simulink model "ExoskeletonControlModel"  (R2022b)
settings: Solver=ode3  StartTime=0.0  StopTime=inf  FixedStep=Ts  RelTol=1e-3
PreLoadFcn:
  | Ts_IO204 = 0.001;
  | 
  | if ~exist('Ts', 'var')
  | Ts = 0.001;
  | end
  | if ~exist('FPGA_Frequency', 'var')
  | FPGA_Frequency = 75000000;
  | end
  | 
  | ts_IO612 = 1e-3;
  | 
  | load('TargetReached.mat')
  | load('ActualPos_inc.mat')
model workspace (MAT data in the model file):
  DeltaData : timeseries (value not decoded)
  EC45_deg2incs = 2276
  EC60_deg2inc = 5461
  EC90_deg2incs = 7111
  Enc2rad_18bit = 2.3968e-05
  Enc2rad_19bit = 1.1984e-05
  Enc2rad_20bit = 5.9921e-06
  GiulioModel : robotics.RigidBodyTree (value not decoded)
  Giulio_Spheric_model : robotics.RigidBodyTree (value not decoded)
  Offset1_ticks = 571315
  Offset2_ticks = 590938.9928
  Offset3_ticks = 457912.8279
  Offset4_ticks = 482293.9763
  Offset5_ticks = 598735.9316
  Offset_M1 = 1.12645499896
  Offset_M2 = 4.02728553608
  Offset_M3 = 5.48587511336
  Offset_M4 = 2.03717511516
  Offset_M5 = 4.4996674016
  T1_Nm : object (value not decoded)
  T2_Nm : object (value not decoded)
  TBmodel : robotics.RigidBodyTree (value not decoded)
  Ts = 0.002
  Xg : object (value not decoded)
  Yg : object (value not decoded)
  Zg : object (value not decoded)
  a2 = 0.27
  change_variable = 0
  d1 = [0 0 0 0 0 0 0 0 0 0 0 0 ... (30001 elements, 30001x1)]
  d1_1 = 0.21074
  d2 = [0 0 0 0 0 0 0 0 0 0 0 0 ... (30001 elements, 30001x1)]
  d2_1 = 0.04864
  d3 = [0 0 0 0 0 0 0 0 0 0 0 0 ... (30001 elements, 30001x1)]
  d4 = [0 0 0 0 0 0 0 0 0 0 0 0 ... (30001 elements, 30001x1)]
  d5 = [0 0 0 0 0 0 0 0 0 0 0 0 ... (30001 elements, 30001x1)]
  d6 = [0 0 0 0 0 0 0 0 0 0 0 0 ... (30001 elements, 30001x1)]
  ee_x = -0.2852
  ee_y = -0.3683
  ee_z = -0.0386
  enc2rad_EC45 = 7.6699e-06
  enc2rad_EC90 = 2.3969e-05
  k1_Nm_ticks = 0.00923
  k2_Nm_ticks = 0.0257
  k3_Nm_ticks = 0.00692
  k4_Nm_ticks = 0.00729
  k5_Nm_ticks = 0.00641
  lower_lim_m1 = -330000
  lower_lim_m2 = -235302
  lower_lim_m3 = -132865
  lower_lim_m4 = -152732
  lower_lim_m5 = -138363
  lower_lim_m6 = -200325
  m1 = 2.441408578
  m2 = 3.750007
  m3 = 1.56250298
  m4 = 1.56250298
  m5 = 1.56250298
  m6 = 1.56250298
  n_oversampling = 8
  offset_sea_1 = 0.5547
  offset_sea_2 = 2.8595
  offset_sea_3 = 3.5058
  offset_sea_4 = 2.8586
  offset_sea_5 = 2.8736
  params : AKSIM (value not decoded)
  pos_th_neg = -180000
  pos_th_pos = 180000
  q1 = -1819347
  q2 = -196752
  q3 = -596465
  q4 = -556807
  q5 = -573932
  q6 = -489063
  sine = [0 0.187999937334 0.751998997352 1.69199492401 3.0079839574 4.6999608335 6.76791878442 9.21184953835 12.0317433196 15.2275888485 18.7993733417 22.7470825122 ... (12501 elements, 12501x1)]
  start : object (value not decoded)
  switch_admittance = 1
  t1 : object (value not decoded)
  t2 : object (value not decoded)
  torsionalStiffnes_M1 = 384.88
  torsionalStiffnes_M2 = 1500
  torsionalStiffnes_M3 = 901.97
  torsionalStiffnes_M4 = 950.86
  torsionalStiffnes_M5 = 930
  torsionalStiffnes_M6 = 914
  upper_lim_m1 = 340000
  upper_lim_m2 = 95467
  upper_lim_m3 = 164951
  upper_lim_m4 = 210607
  upper_lim_m5 = 252595
  upper_lim_m6 = 96694
  vel_th_neg = -100
  vel_th_pos = 100
  x = 0
undefined symbols (not defined in the file): C, DiscIntNeverNeededParam
libraries: canmsglib x285, speedgoatlib_IO614 x245, simulink x26, slrealtimeloglib x9, simulink_extras x6, robotmaniplib x6
(part 4 of 13)

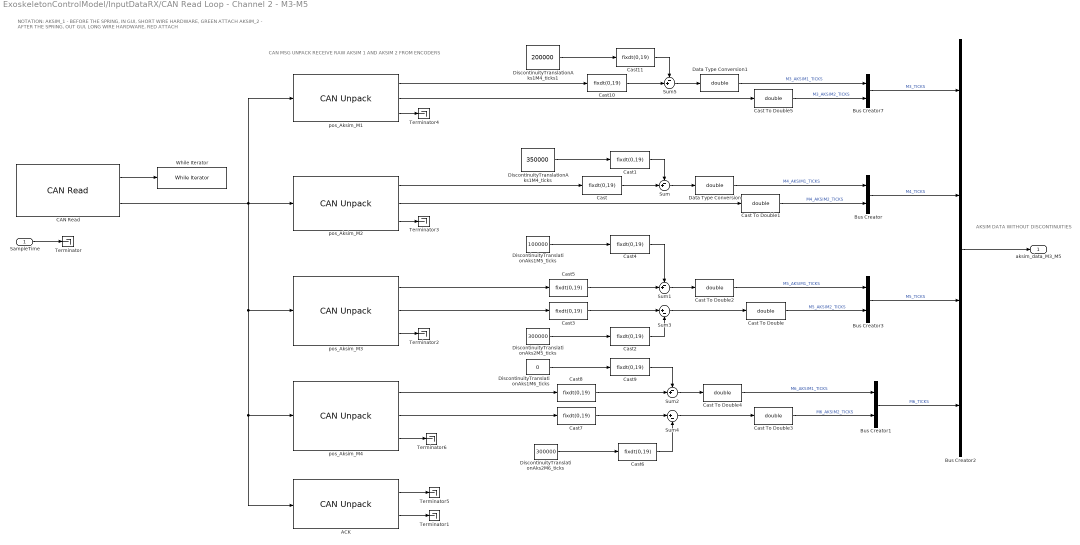
== system ExoskeletonControlModel/InputDataRX/CAN Read Loop - Channel 2 - M3-M5 ==
  note: AKSIM DATA WITHOUT DISCONTINUITIES
  note: CAN MSG UNPACK
      | RECEIVE RAW AKSIM 1 AND AKSIM 2 FROM ENCODERS
  note: NOTATION:
      | AKSIM_1 - BEFORE THE SPRING, IN GUI, SHORT WIRE HARDWARE, GREEN ATTACH
      | AKSIM_2 - AFTER THE SPRING, OUT GUI, LONG WIRE HARDWARE, RED ATTACH
  SampleTime : Inport
  ACK : canmsglib/CAN Unpack  MsgList=(none)  MsgName=CAN Msg  MsgIDType=Standard (11-bit identifier)  MsgIdentifier=hex2dec('10C')  MsgLength=8  SignalInfo={ 'Signal1', '0', '8', 'LE', 'signed', 'Standard', '0', '1', '0', '-Inf', 'Inf' }  IDPort=off  TimestampPort=off  ErrorPort=off  RemotePort=off  LengthPort=off  StatusPort=on  ApplyMinMax=off
  Bus Creator{,1,3,7} (4 alike) : BusCreator  Inputs=2
  Bus Creator2 : BusCreator  Inputs=4
  CAN Read : speedgoatlib_IO614/CAN/CAN Read  id=1  sampleTime=-1  portSelection=2  messageType=CAN  protl=IO614  ptIdx=1  isFDMod=0
  Cast{,1..11} (12 alike) : DataTypeConversion  OutMin=0  OutMax=2^19-1  OutDataTypeStr=fixdt(0,19)  SaturateOnIntegerOverflow=off  RndMeth=Floor
  Cast To Double{,1..5} (6 alike) : DataTypeConversion  OutDataTypeStr=double  SaturateOnIntegerOverflow=off  RndMeth=Floor
  Data Type Conversion : DataTypeConversion  OutDataTypeStr=double  SaturateOnIntegerOverflow=off  RndMeth=Floor
  Data Type Conversion1 : DataTypeConversion  OutDataTypeStr=double  SaturateOnIntegerOverflow=off  RndMeth=Floor
  DiscontinuityTranslationAks1M4_ticks : Constant  Value=350000
  DiscontinuityTranslationAks1M4_ticks1 : Constant  Value=200000
  DiscontinuityTranslationAks1M5_ticks : Constant  Value=100000
  DiscontinuityTranslationAks1M6_ticks : Constant  Value=0
  DiscontinuityTranslationAks2M5_ticks : Constant  Value=300000
  DiscontinuityTranslationAks2M6_ticks : Constant  Value=300000
  Sum{,1..2,5} (4 alike) : Sum  Inputs=-+|  OutDataTypeStr=Inherit: Same as first input
  Sum3 : Sum  Inputs=|+-  OutDataTypeStr=Inherit: Same as first input
  Sum4 : Sum  Inputs=|+-  OutDataTypeStr=Inherit: Same as first input
  Terminator{,1..6} (7 alike) : Terminator
  While Iterator : WhileIterator  MaxIters=501  WhileBlockType=do-while
  pos_Aksim_M1 : canmsglib/CAN Unpack  MsgList=(none)  MsgName=CAN Msg  MsgIDType=Standard (11-bit identifier)  MsgIdentifier=hex2dec('102')  MsgLength=8  SignalInfo={ 'AKSIM_1', '0', '32', 'LE', 'unsigned', 'Standard', '0', '1', '0', '-Inf', 'Inf'; 'AKSIM_2', '32', '32', 'LE', 'unsigned', 'Standard', '0', '1', '0', '-Inf', 'Inf' }  IDPort=off  TimestampPort=off  ErrorPort=off  RemotePort=on  LengthPort=off  StatusPort=off  ApplyMinMax=off
  pos_Aksim_M2 : canmsglib/CAN Unpack  MsgList=(none)  MsgName=CAN Msg  MsgIDType=Standard (11-bit identifier)  MsgIdentifier=hex2dec('202')  MsgLength=8  SignalInfo={ 'AKSIM_1', '0', '32', 'LE', 'unsigned', 'Standard', '0', '1', '0', '-Inf', 'Inf'; 'AKSIM_2', '32', '32', 'LE', 'unsigned', 'Standard', '0', '1', '0', '-Inf', 'Inf' }  IDPort=off  TimestampPort=off  ErrorPort=off  RemotePort=on  LengthPort=off  StatusPort=off  ApplyMinMax=off
  pos_Aksim_M3 : canmsglib/CAN Unpack  MsgList=(none)  MsgName=CAN Msg  MsgIDType=Standard (11-bit identifier)  MsgIdentifier=hex2dec('302')  MsgLength=8  SignalInfo={ 'AKSIM_1', '0', '32', 'LE', 'unsigned', 'Standard', '0', '1', '0', '-Inf', 'Inf'; 'AKSIM_2', '32', '32', 'LE', 'unsigned', 'Standard', '0', '1', '0', '-Inf', 'Inf' }  IDPort=off  TimestampPort=off  ErrorPort=off  RemotePort=on  LengthPort=off  StatusPort=off  ApplyMinMax=off
  pos_Aksim_M4 : canmsglib/CAN Unpack  MsgList=(none)  MsgName=CAN Msg  MsgIDType=Standard (11-bit identifier)  MsgIdentifier=hex2dec('402')  MsgLength=8  SignalInfo={ 'AKSIM_1', '0', '32', 'LE', 'unsigned', 'Standard', '0', '1', '0', '-Inf', 'Inf'; 'AKSIM_2', '32', '32', 'LE', 'unsigned', 'Standard', '0', '1', '0', '-Inf', 'Inf' }  IDPort=off  TimestampPort=off  ErrorPort=off  RemotePort=on  LengthPort=off  StatusPort=off  ApplyMinMax=off
  aksim_data_M3_M5 : Outport
  wires:
  SampleTime/1 -> Terminator/1
  CAN Read/1 -> While Iterator/1
  pos_Aksim_M1/3 -> Terminator4/1
  Cast To Double5/1 -> Bus Creator7/2  "M3_AKSIM2_TICKS"
  ACK/2 -> Terminator1/1
  pos_Aksim_M2/1 -> Cast/1
  ACK/1 -> Terminator5/1
  Data Type Conversion1/1 -> Bus Creator7/1  "M3_AKSIM1_TICKS"
  pos_Aksim_M2/3 -> Terminator3/1
  Bus Creator2/1 -> aksim_data_M3_M5/1
  Bus Creator/1 -> Bus Creator2/2  "M4_TICKS"
  Bus Creator7/1 -> Bus Creator2/1  "M3_TICKS"
  pos_Aksim_M3/1 -> Cast5/1
  Bus Creator3/1 -> Bus Creator2/3  "M5_TICKS"
  pos_Aksim_M3/2 -> Cast3/1
  pos_Aksim_M3/3 -> Terminator2/1
  Sum/1 -> Data Type Conversion/1
  pos_Aksim_M2/2 -> Cast To Double1/1
  Sum3/1 -> Cast To Double/1
  Cast3/1 -> Sum3/1
  DiscontinuityTranslationAks2M5_ticks/1 -> Cast2/1
  DiscontinuityTranslationAks1M4_ticks/1 -> Cast1/1
  Cast/1 -> Sum/2
  Cast1/1 -> Sum/1
  Cast To Double/1 -> Bus Creator3/2  "M5_AKSIM2_TICKS"
  Cast To Double1/1 -> Bus Creator/2  "M4_AKSIM2_TICKS"
  Data Type Conversion/1 -> Bus Creator/1  "M4_AKSIM1_TICKS"
  Cast2/1 -> Sum3/2
  Cast To Double2/1 -> Bus Creator3/1  "M5_AKSIM1_TICKS"
  Sum1/1 -> Cast To Double2/1
  DiscontinuityTranslationAks1M5_ticks/1 -> Cast4/1
  Cast5/1 -> Sum1/2
  Cast4/1 -> Sum1/1
  Cast9/1 -> Sum2/1
  Cast6/1 -> Sum4/2
  Cast8/1 -> Sum2/2
  DiscontinuityTranslationAks1M6_ticks/1 -> Cast9/1
  Cast To Double4/1 -> Bus Creator1/1  "M6_AKSIM1_TICKS"
  Cast To Double3/1 -> Bus Creator1/2  "M6_AKSIM2_TICKS"
  Sum4/1 -> Cast To Double3/1
  DiscontinuityTranslationAks2M6_ticks/1 -> Cast6/1
  pos_Aksim_M4/1 -> Cast8/1
  pos_Aksim_M4/2 -> Cast7/1
  Sum2/1 -> Cast To Double4/1
  Cast7/1 -> Sum4/1
  CAN Read/2 -> pos_Aksim_M3/1, ACK/1, pos_Aksim_M4/1, pos_Aksim_M2/1, pos_Aksim_M1/1
  pos_Aksim_M4/3 -> Terminator6/1
  Bus Creator1/1 -> Bus Creator2/4  "M6_TICKS"
  Cast11/1 -> Sum5/1
  Sum5/1 -> Data Type Conversion1/1
  Cast10/1 -> Sum5/2
  DiscontinuityTranslationAks1M4_ticks1/1 -> Cast11/1
  pos_Aksim_M1/1 -> Cast10/1
  pos_Aksim_M1/2 -> Cast To Double5/1

== system ExoskeletonControlModel/InputDataRX/CAN Read Loop - Channel 3 ==
  note: PDO M1
  note: PDO M2
  note: STATUS MODE M1 M2
  note: CAN MSG FROM EPOS M1 M2
  SampleTime : Inport
  Bus Creator1 : BusCreator  Inputs=3
  Bus Creator2 : BusCreator  Inputs=5
  Bus Creator3 : BusCreator  Inputs=5
  Bus Creator4 : BusCreator  Inputs=9
  Bus Creator5 : BusCreator  Inputs=4
  Bus Creator6 : BusCreator  Inputs=3
  CAN Read : speedgoatlib_IO614/CAN/CAN Read  id=1  sampleTime=-1  portSelection=3  messageType=CAN  protl=IO614  ptIdx=2  isFDMod=0
  Constant : Constant
  Constant1 : Constant
  EMCY : canmsglib/CAN Unpack  MsgList=(none)  MsgName=CAN Msg  MsgIDType=Standard (11-bit identifier)  MsgIdentifier=129  MsgLength=8  SignalInfo={ 'ErrorCode', '0', '16', 'LE', 'unsigned', 'Standard', '0', '1', '0', '-Inf', 'Inf'; 'ErrorReg', '16', '8', 'LE', 'unsigned', 'Standard', '0', '1', '0', '-Inf', 'Inf' }  IDPort=off  TimestampPort=off  ErrorPort=off  RemotePort=off  LengthPort=off  StatusPort=off  ApplyMinMax=off
  EMCY_m2 : canmsglib/CAN Unpack  MsgList=(none)  MsgName=CAN Msg  MsgIDType=Standard (11-bit identifier)  MsgIdentifier=130  MsgLength=8  SignalInfo={ 'ErrorCode', '0', '16', 'LE', 'unsigned', 'Standard', '0', '1', '0', '-Inf', 'Inf'; 'ErrorReg', '16', '8', 'LE', 'unsigned', 'Standard', '0', '1', '0', '-Inf', 'Inf' }  IDPort=off  TimestampPort=off  ErrorPort=off  RemotePort=off  LengthPort=off  StatusPort=off  ApplyMinMax=off
  HEARTBEAT : canmsglib/CAN Unpack  MsgList=(none)  MsgName=CAN Msg  MsgIDType=Standard (11-bit identifier)  MsgIdentifier=hex2dec('701')  MsgLength=1  SignalInfo={ 'NMT_state', '0', '8', 'LE', 'unsigned', 'Standard', '0', '1', '0', '-Inf', 'Inf' }  IDPort=off  TimestampPort=off  ErrorPort=off  RemotePort=off  LengthPort=off  StatusPort=off  ApplyMinMax=off
  HEARTBEAT_m2 : canmsglib/CAN Unpack  MsgList=(none)  MsgName=CAN Msg  MsgIDType=Standard (11-bit identifier)  MsgIdentifier=hex2dec('702')  MsgLength=1  SignalInfo={ 'NMT_state', '0', '8', 'LE', 'unsigned', 'Standard', '0', '1', '0', '-Inf', 'Inf' }  IDPort=off  TimestampPort=off  ErrorPort=off  RemotePort=off  LengthPort=off  StatusPort=off  ApplyMinMax=off
  Terminator : Terminator
  Terminator1 : Terminator
  Terminator2 : Terminator
  TxPDO1 : canmsglib/CAN Unpack  MsgList=(none)  MsgName=CAN Msg  MsgIDType=Standard (11-bit identifier)  MsgIdentifier=hex2dec('181')  MsgLength=7  SignalInfo={ 'Statusword', '0', '16', 'LE', 'unsigned', 'Standard', '0', '1', '0', '-Inf', 'Inf'; 'Modes Operation', '16', '8', 'LE', 'unsigned', 'Standard', '0', '1', '0', '-Inf', 'Inf'; 'Current actual', '24', '32', 'LE', 'signed', 'Standard', '0', '1', '0', '-Inf', 'Inf' }  IDPort=off  TimestampPort=off  ErrorPort=off  RemotePort=off  LengthPort=off  StatusPort=off  ApplyMinMax=off
  TxPDO1_m2 : canmsglib/CAN Unpack  MsgList=(none)  MsgName=CAN Msg  MsgIDType=Standard (11-bit identifier)  MsgIdentifier=hex2dec('182')  MsgLength=7  SignalInfo={ 'Statusword', '0', '16', 'LE', 'unsigned', 'Standard', '0', '1', '0', '-Inf', 'Inf'; 'Modes Operation', '16', '8', 'LE', 'unsigned', 'Standard', '0', '1', '0', '-Inf', 'Inf'; 'Current actual', '24', '32', 'LE', 'signed', 'Standard', '0', '1', '0', '-Inf', 'Inf' }  IDPort=off  TimestampPort=off  ErrorPort=off  RemotePort=off  LengthPort=off  StatusPort=off  ApplyMinMax=off
  TxPDO2 : canmsglib/CAN Unpack  MsgList=(none)  MsgName=CAN Msg  MsgIDType=Standard (11-bit identifier)  MsgIdentifier=hex2dec('281')  MsgLength=4  SignalInfo={ 'Pos Actual', '0', '32', 'LE', 'signed', 'Standard', '0', '1', '0', '-Inf', 'Inf' }  IDPort=off  TimestampPort=off  ErrorPort=off  RemotePort=off  LengthPort=off  StatusPort=off  ApplyMinMax=off
  TxPDO2_m2 : canmsglib/CAN Unpack  MsgList=(none)  MsgName=CAN Msg  MsgIDType=Standard (11-bit identifier)  MsgIdentifier=hex2dec('282')  MsgLength=4  SignalInfo={ 'Pos Actual', '0', '32', 'LE', 'signed', 'Standard', '0', '1', '0', '-Inf', 'Inf' }  IDPort=off  TimestampPort=off  ErrorPort=off  RemotePort=off  LengthPort=off  StatusPort=off  ApplyMinMax=off
  TxPDO4 : canmsglib/CAN Unpack  MsgList=(none)  MsgName=CAN Msg  MsgIDType=Standard (11-bit identifier)  MsgIdentifier=hex2dec('481')  MsgLength=8  SignalInfo={ 'Velocity Actual Value', '0', '32', 'LE', 'signed', 'Standard', '0', '1', '0', '-Inf', 'Inf'; 'Torque Actual', '32', '16', 'LE', 'signed', 'Standard', '0', '1', '0', '-Inf', 'Inf'; 'Torque Actual Averaged', '48', '16', 'LE', 'signed', 'Standard', '0', '1', '0', '-Inf', 'Inf' }  IDPort=off  TimestampPort=off  ErrorPort=off  RemotePort=off  LengthPort=off  StatusPort=off  ApplyMinMax=off
  TxPDO4_m2 : canmsglib/CAN Unpack  MsgList=(none)  MsgName=CAN Msg  MsgIDType=Standard (11-bit identifier)  MsgIdentifier=hex2dec('482')  MsgLength=8  SignalInfo={ 'Velocity Actual Value', '0', '32', 'LE', 'signed', 'Standard', '0', '1', '0', '-Inf', 'Inf'; 'Torque Actual', '32', '16', 'LE', 'signed', 'Standard', '0', '1', '0', '-Inf', 'Inf'; 'Torque Actual Averaged', '48', '16', 'LE', 'signed', 'Standard', '0', '1', '0', '-Inf', 'Inf' }  IDPort=off  TimestampPort=off  ErrorPort=off  RemotePort=off  LengthPort=off  StatusPort=off  ApplyMinMax=off
  While Iterator : WhileIterator  MaxIters=501  WhileBlockType=do-while
  txSDO : canmsglib/CAN Unpack  MsgList=(none)  MsgName=CAN Msg  MsgIDType=Standard (11-bit identifier)  MsgIdentifier=1409  MsgLength=8  SignalInfo={ 'data', '32', '32', 'LE', 'signed', 'Standard', '0', '1', '0', '-Inf', 'Inf'; 'Index', '8', '16', 'LE', 'unsigned', 'Standard', '0', '1', '0', '-Inf', 'Inf'; 'SubIndex', '24', '8', 'LE', 'unsigned', 'Standard', '0', '1', '0', '-Inf', 'Inf' }  IDPort=off  TimestampPort=off  ErrorPort=off  RemotePort=off  LengthPort=off  StatusPort=off  ApplyMinMax=off
  txSDO1 : canmsglib/CAN Unpack  MsgList=(none)  MsgName=CAN Msg  MsgIDType=Standard (11-bit identifier)  MsgIdentifier=1410  MsgLength=8  SignalInfo={ 'data', '32', '32', 'LE', 'signed', 'Standard', '0', '1', '0', '-Inf', 'Inf'; 'Index', '8', '16', 'LE', 'unsigned', 'Standard', '0', '1', '0', '-Inf', 'Inf'; 'SubIndex', '24', '8', 'LE', 'unsigned', 'Standard', '0', '1', '0', '-Inf', 'Inf' }  IDPort=off  TimestampPort=off  ErrorPort=off  RemotePort=off  LengthPort=off  StatusPort=off  ApplyMinMax=off
  txSDO2 : canmsglib/CAN Unpack  MsgList=(none)  MsgName=CAN Msg  MsgIDType=Standard (11-bit identifier)  MsgIdentifier=1411  MsgLength=8  SignalInfo={ 'data', '32', '32', 'LE', 'signed', 'Standard', '0', '1', '0', '-Inf', 'Inf'; 'Index', '8', '16', 'LE', 'unsigned', 'Standard', '0', '1', '0', '-Inf', 'Inf'; 'SubIndex', '24', '8', 'LE', 'unsigned', 'Standard', '0', '1', '0', '-Inf', 'Inf' }  IDPort=off  TimestampPort=off  ErrorPort=off  RemotePort=off  LengthPort=off  StatusPort=off  ApplyMinMax=off
  SDOs : Outport
  emcy : Outport  Port=2
  NMT_state : Outport  Port=3
  status_mode_m1_m2 : Outport  Port=4
  PDO_m1 : Outport  Port=5
  PDO_m2 : Outport  Port=6
  wires:
  SampleTime/1 -> Terminator/1
  Bus Creator4/1 -> SDOs/1
  txSDO/3 -> Bus Creator4/3  "SDO_subIndex"
  EMCY/2 -> Terminator1/1
  EMCY/1 -> Bus Creator1/1  "error_code_m1"
  Bus Creator1/1 -> emcy/1
  HEARTBEAT/1 -> Bus Creator6/1  "NMT_state_1"
  txSDO/1 -> Bus Creator4/1  "SDO_data"
  txSDO/2 -> Bus Creator4/2  "SDO_index"
  TxPDO1/1 -> Bus Creator5/1  "statusword_1"
  TxPDO1/2 -> Bus Creator5/2  "mode_1"
  TxPDO1/3 -> Bus Creator2/1  "current_actual_1"
  TxPDO2/1 -> Bus Creator2/2  "pos_actual_1"
  TxPDO4/1 -> Bus Creator2/3  "velocity_actual_1"
  TxPDO4/2 -> Bus Creator2/4  "torque_actual_1"
  TxPDO1_m2/3 -> Bus Creator3/1  "current_actual_2"
  TxPDO4_m2/2 -> Bus Creator3/4  "torque_actual_2"
  TxPDO4_m2/1 -> Bus Creator3/3  "velocity_actual_2"
  TxPDO1_m2/2 -> Bus Creator5/4  "mode_2"
  TxPDO2_m2/1 -> Bus Creator3/2  "pos_actual_2"
  TxPDO1_m2/1 -> Bus Creator5/3  "statusword_2"
  Bus Creator2/1 -> PDO_m1/1
  Bus Creator3/1 -> PDO_m2/1
  Bus Creator5/1 -> status_mode_m1_m2/1
  EMCY_m2/1 -> Bus Creator1/2  "error_code_m2"
  EMCY_m2/2 -> Terminator2/1
  HEARTBEAT_m2/1 -> Bus Creator6/2  "NMT_state_2"
  Bus Creator6/1 -> NMT_state/1
  TxPDO4/3 -> Bus Creator2/5  "torque_averaged_1"
  TxPDO4_m2/3 -> Bus Creator3/5  "torque_averaged_2"
  txSDO1/1 -> Bus Creator4/4  "SDO_data2"
  txSDO1/2 -> Bus Creator4/5  "SDO_index2"
  txSDO1/3 -> Bus Creator4/6  "SDO_subIndex2"
  txSDO2/2 -> Bus Creator4/8  "SDO_index3"
  txSDO2/3 -> Bus Creator4/9  "SDO_subIndex3"
  txSDO2/1 -> Bus Creator4/7  "SDO_data3"
  CAN Read/1 -> While Iterator/1
  CAN Read/2 -> txSDO/1, txSDO1/1, txSDO2/1, EMCY_m2/1, HEARTBEAT_m2/1, TxPDO1/1, TxPDO2/1, TxPDO4/1, TxPDO1_m2/1, TxPDO2_m2/1, TxPDO4_m2/1, HEARTBEAT/1, EMCY/1
  Constant/1 -> Bus Creator1/3  "future"
  Constant1/1 -> Bus Creator6/3  "future_NMT"

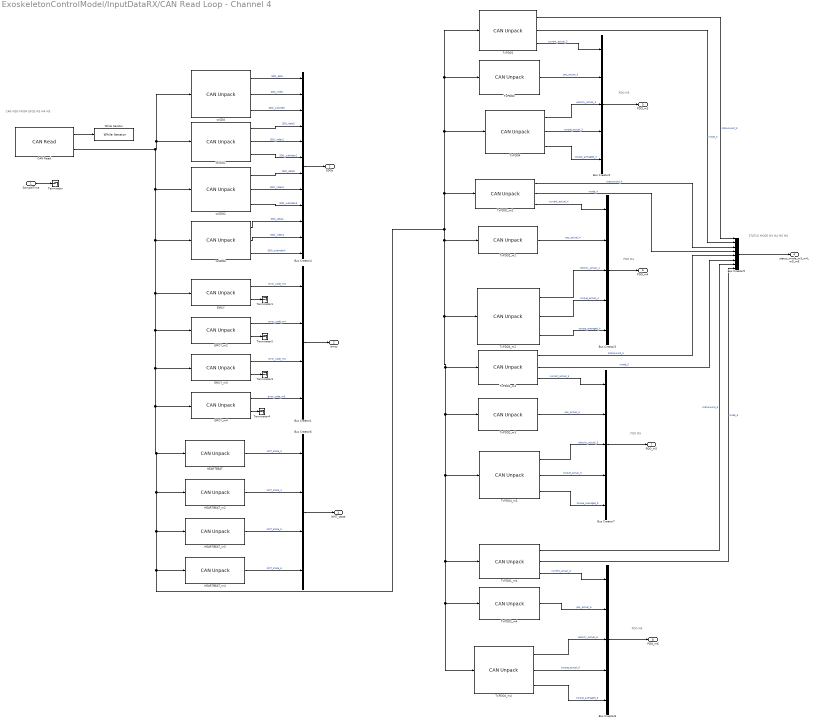
== system ExoskeletonControlModel/InputDataRX/CAN Read Loop - Channel 4 ==
  note: STATUS MODE M3 M4 M5 M6
  note: CAN MSG FROM EPOS M3 M4 M5
  note: PDO M3
  note: PDO M5
  note: PDO M4
  note: PDO M6
  SampleTime : Inport
  Bus Creator1 : BusCreator  Inputs=4
  Bus Creator{2..3,7..8} (4 alike) : BusCreator  Inputs=5
  Bus Creator4 : BusCreator  Inputs=12
  Bus Creator5 : BusCreator  Inputs=8
  Bus Creator6 : BusCreator  Inputs=4
  CAN Read : speedgoatlib_IO614/CAN/CAN Read  id=1  sampleTime=-1  portSelection=4  messageType=CAN  protl=IO614  ptIdx=3  isFDMod=0
  EMCY : canmsglib/CAN Unpack  MsgList=(none)  MsgName=CAN Msg  MsgIDType=Standard (11-bit identifier)  MsgIdentifier=129  MsgLength=8  SignalInfo={ 'ErrorCode', '0', '16', 'LE', 'unsigned', 'Standard', '0', '1', '0', '-Inf', 'Inf'; 'ErrorReg', '16', '8', 'LE', 'unsigned', 'Standard', '0', '1', '0', '-Inf', 'Inf' }  IDPort=off  TimestampPort=off  ErrorPort=off  RemotePort=off  LengthPort=off  StatusPort=off  ApplyMinMax=off
  EMCY_m2 : canmsglib/CAN Unpack  MsgList=(none)  MsgName=CAN Msg  MsgIDType=Standard (11-bit identifier)  MsgIdentifier=130  MsgLength=8  SignalInfo={ 'ErrorCode', '0', '16', 'LE', 'unsigned', 'Standard', '0', '1', '0', '-Inf', 'Inf'; 'ErrorReg', '16', '8', 'LE', 'unsigned', 'Standard', '0', '1', '0', '-Inf', 'Inf' }  IDPort=off  TimestampPort=off  ErrorPort=off  RemotePort=off  LengthPort=off  StatusPort=off  ApplyMinMax=off
  EMCY_m3 : canmsglib/CAN Unpack  MsgList=(none)  MsgName=CAN Msg  MsgIDType=Standard (11-bit identifier)  MsgIdentifier=131  MsgLength=8  SignalInfo={ 'ErrorCode', '0', '16', 'LE', 'unsigned', 'Standard', '0', '1', '0', '-Inf', 'Inf'; 'ErrorReg', '16', '8', 'LE', 'unsigned', 'Standard', '0', '1', '0', '-Inf', 'Inf' }  IDPort=off  TimestampPort=off  ErrorPort=off  RemotePort=off  LengthPort=off  StatusPort=off  ApplyMinMax=off
  EMCY_m4 : canmsglib/CAN Unpack  MsgList=(none)  MsgName=CAN Msg  MsgIDType=Standard (11-bit identifier)  MsgIdentifier=132  MsgLength=8  SignalInfo={ 'ErrorCode', '0', '16', 'LE', 'unsigned', 'Standard', '0', '1', '0', '-Inf', 'Inf'; 'ErrorReg', '16', '8', 'LE', 'unsigned', 'Standard', '0', '1', '0', '-Inf', 'Inf' }  IDPort=off  TimestampPort=off  ErrorPort=off  RemotePort=off  LengthPort=off  StatusPort=off  ApplyMinMax=off
  HEARTBEAT : canmsglib/CAN Unpack  MsgList=(none)  MsgName=CAN Msg  MsgIDType=Standard (11-bit identifier)  MsgIdentifier=hex2dec('701')  MsgLength=1  SignalInfo={ 'NMT_state', '0', '8', 'LE', 'unsigned', 'Standard', '0', '1', '0', '-Inf', 'Inf' }  IDPort=off  TimestampPort=off  ErrorPort=off  RemotePort=off  LengthPort=off  StatusPort=off  ApplyMinMax=off
  HEARTBEAT_m2 : canmsglib/CAN Unpack  MsgList=(none)  MsgName=CAN Msg  MsgIDType=Standard (11-bit identifier)  MsgIdentifier=hex2dec('702')  MsgLength=1  SignalInfo={ 'NMT_state', '0', '8', 'LE', 'unsigned', 'Standard', '0', '1', '0', '-Inf', 'Inf' }  IDPort=off  TimestampPort=off  ErrorPort=off  RemotePort=off  LengthPort=off  StatusPort=off  ApplyMinMax=off
  HEARTBEAT_m3 : canmsglib/CAN Unpack  MsgList=(none)  MsgName=CAN Msg  MsgIDType=Standard (11-bit identifier)  MsgIdentifier=hex2dec('703')  MsgLength=1  SignalInfo={ 'NMT_state', '0', '8', 'LE', 'unsigned', 'Standard', '0', '1', '0', '-Inf', 'Inf' }  IDPort=off  TimestampPort=off  ErrorPort=off  RemotePort=off  LengthPort=off  StatusPort=off  ApplyMinMax=off
  HEARTBEAT_m4 : canmsglib/CAN Unpack  MsgList=(none)  MsgName=CAN Msg  MsgIDType=Standard (11-bit identifier)  MsgIdentifier=hex2dec('704')  MsgLength=1  SignalInfo={ 'NMT_state', '0', '8', 'LE', 'unsigned', 'Standard', '0', '1', '0', '-Inf', 'Inf' }  IDPort=off  TimestampPort=off  ErrorPort=off  RemotePort=off  LengthPort=off  StatusPort=off  ApplyMinMax=off
  Terminator{,1..4} (5 alike) : Terminator
  TxPDO1 : canmsglib/CAN Unpack  MsgList=(none)  MsgName=CAN Msg  MsgIDType=Standard (11-bit identifier)  MsgIdentifier=hex2dec('181')  MsgLength=7  SignalInfo={ 'Statusword', '0', '16', 'LE', 'unsigned', 'Standard', '0', '1', '0', '-Inf', 'Inf'; 'Modes Operation', '16', '8', 'LE', 'unsigned', 'Standard', '0', '1', '0', '-Inf', 'Inf'; 'Current actual', '24', '32', 'LE', 'signed', 'Standard', '0', '1', '0', '-Inf', 'Inf' }  IDPort=off  TimestampPort=off  ErrorPort=off  RemotePort=off  LengthPort=off  StatusPort=off  ApplyMinMax=off
  TxPDO1_m2 : canmsglib/CAN Unpack  MsgList=(none)  MsgName=CAN Msg  MsgIDType=Standard (11-bit identifier)  MsgIdentifier=hex2dec('182')  MsgLength=7  SignalInfo={ 'Statusword', '0', '16', 'LE', 'unsigned', 'Standard', '0', '1', '0', '-Inf', 'Inf'; 'Modes Operation', '16', '8', 'LE', 'unsigned', 'Standard', '0', '1', '0', '-Inf', 'Inf'; 'Current actual', '24', '32', 'LE', 'signed', 'Standard', '0', '1', '0', '-Inf', 'Inf' }  IDPort=off  TimestampPort=off  ErrorPort=off  RemotePort=off  LengthPort=off  StatusPort=off  ApplyMinMax=off
  TxPDO1_m3 : canmsglib/CAN Unpack  MsgList=(none)  MsgName=CAN Msg  MsgIDType=Standard (11-bit identifier)  MsgIdentifier=hex2dec('183')  MsgLength=7  SignalInfo={ 'Statusword', '0', '16', 'LE', 'unsigned', 'Standard', '0', '1', '0', '-Inf', 'Inf'; 'Modes Operation', '16', '8', 'LE', 'unsigned', 'Standard', '0', '1', '0', '-Inf', 'Inf'; 'Current actual', '24', '32', 'LE', 'signed', 'Standard', '0', '1', '0', '-Inf', 'Inf' }  IDPort=off  TimestampPort=off  ErrorPort=off  RemotePort=off  LengthPort=off  StatusPort=off  ApplyMinMax=off
  TxPDO1_m4 : canmsglib/CAN Unpack  MsgList=(none)  MsgName=CAN Msg  MsgIDType=Standard (11-bit identifier)  MsgIdentifier=hex2dec('184')  MsgLength=7  SignalInfo={ 'Statusword', '0', '16', 'LE', 'unsigned', 'Standard', '0', '1', '0', '-Inf', 'Inf'; 'Modes Operation', '16', '8', 'LE', 'unsigned', 'Standard', '0', '1', '0', '-Inf', 'Inf'; 'Current actual', '24', '32', 'LE', 'signed', 'Standard', '0', '1', '0', '-Inf', 'Inf' }  IDPort=off  TimestampPort=off  ErrorPort=off  RemotePort=off  LengthPort=off  StatusPort=off  ApplyMinMax=off
  TxPDO2 : canmsglib/CAN Unpack  MsgList=(none)  MsgName=CAN Msg  MsgIDType=Standard (11-bit identifier)  MsgIdentifier=hex2dec('281')  MsgLength=4  SignalInfo={ 'Pos Actual', '0', '32', 'LE', 'signed', 'Standard', '0', '1', '0', '-Inf', 'Inf' }  IDPort=off  TimestampPort=off  ErrorPort=off  RemotePort=off  LengthPort=off  StatusPort=off  ApplyMinMax=off
  TxPDO2_m2 : canmsglib/CAN Unpack  MsgList=(none)  MsgName=CAN Msg  MsgIDType=Standard (11-bit identifier)  MsgIdentifier=hex2dec('282')  MsgLength=4  SignalInfo={ 'Pos Actual', '0', '32', 'LE', 'signed', 'Standard', '0', '1', '0', '-Inf', 'Inf' }  IDPort=off  TimestampPort=off  ErrorPort=off  RemotePort=off  LengthPort=off  StatusPort=off  ApplyMinMax=off
  TxPDO2_m3 : canmsglib/CAN Unpack  MsgList=(none)  MsgName=CAN Msg  MsgIDType=Standard (11-bit identifier)  MsgIdentifier=hex2dec('283')  MsgLength=4  SignalInfo={ 'Pos Actual', '0', '32', 'LE', 'signed', 'Standard', '0', '1', '0', '-Inf', 'Inf' }  IDPort=off  TimestampPort=off  ErrorPort=off  RemotePort=off  LengthPort=off  StatusPort=off  ApplyMinMax=off
  TxPDO2_m4 : canmsglib/CAN Unpack  MsgList=(none)  MsgName=CAN Msg  MsgIDType=Standard (11-bit identifier)  MsgIdentifier=hex2dec('284')  MsgLength=4  SignalInfo={ 'Pos Actual', '0', '32', 'LE', 'signed', 'Standard', '0', '1', '0', '-Inf', 'Inf' }  IDPort=off  TimestampPort=off  ErrorPort=off  RemotePort=off  LengthPort=off  StatusPort=off  ApplyMinMax=off
  TxPDO4 : canmsglib/CAN Unpack  MsgList=(none)  MsgName=CAN Msg  MsgIDType=Standard (11-bit identifier)  MsgIdentifier=hex2dec('481')  MsgLength=8  SignalInfo={ 'Velocity Actual Value', '0', '32', 'LE', 'signed', 'Standard', '0', '1', '0', '-Inf', 'Inf'; 'Torque Actual', '32', '16', 'LE', 'signed', 'Standard', '0', '1', '0', '-Inf', 'Inf'; 'Torque Actual Averaged', '48', '16', 'LE', 'signed', 'Standard', '0', '1', '0', '-Inf', 'Inf' }  IDPort=off  TimestampPort=off  ErrorPort=off  RemotePort=off  LengthPort=off  StatusPort=off  ApplyMinMax=off
  TxPDO4_m2 : canmsglib/CAN Unpack  MsgList=(none)  MsgName=CAN Msg  MsgIDType=Standard (11-bit identifier)  MsgIdentifier=hex2dec('482')  MsgLength=8  SignalInfo={ 'Velocity Actual Value', '0', '32', 'LE', 'signed', 'Standard', '0', '1', '0', '-Inf', 'Inf'; 'Torque Actual', '32', '16', 'LE', 'signed', 'Standard', '0', '1', '0', '-Inf', 'Inf'; 'Torque Actual Averaged', '48', '16', 'LE', 'signed', 'Standard', '0', '1', '0', '-Inf', 'Inf' }  IDPort=off  TimestampPort=off  ErrorPort=off  RemotePort=off  LengthPort=off  StatusPort=off  ApplyMinMax=off
  TxPDO4_m3 : canmsglib/CAN Unpack  MsgList=(none)  MsgName=CAN Msg  MsgIDType=Standard (11-bit identifier)  MsgIdentifier=hex2dec('483')  MsgLength=8  SignalInfo={ 'Velocity Actual Value', '0', '32', 'LE', 'signed', 'Standard', '0', '1', '0', '-Inf', 'Inf'; 'Torque Actual', '32', '16', 'LE', 'signed', 'Standard', '0', '1', '0', '-Inf', 'Inf'; 'Torque Actual Averaged', '48', '16', 'LE', 'signed', 'Standard', '0', '1', '0', '-Inf', 'Inf' }  IDPort=off  TimestampPort=off  ErrorPort=off  RemotePort=off  LengthPort=off  StatusPort=off  ApplyMinMax=off
  TxPDO4_m4 : canmsglib/CAN Unpack  MsgList=(none)  MsgName=CAN Msg  MsgIDType=Standard (11-bit identifier)  MsgIdentifier=hex2dec('484')  MsgLength=8  SignalInfo={ 'Velocity Actual Value', '0', '32', 'LE', 'signed', 'Standard', '0', '1', '0', '-Inf', 'Inf'; 'Torque Actual', '32', '16', 'LE', 'signed', 'Standard', '0', '1', '0', '-Inf', 'Inf'; 'Torque Actual Averaged', '48', '16', 'LE', 'signed', 'Standard', '0', '1', '0', '-Inf', 'Inf' }  IDPort=off  TimestampPort=off  ErrorPort=off  RemotePort=off  LengthPort=off  StatusPort=off  ApplyMinMax=off
  While Iterator : WhileIterator  MaxIters=501  WhileBlockType=do-while
  txSDO : canmsglib/CAN Unpack  MsgList=(none)  MsgName=CAN Msg  MsgIDType=Standard (11-bit identifier)  MsgIdentifier=1409  MsgLength=8  SignalInfo={ 'data', '32', '32', 'LE', 'signed', 'Standard', '0', '1', '0', '-Inf', 'Inf'; 'Index', '8', '16', 'LE', 'unsigned', 'Standard', '0', '1', '0', '-Inf', 'Inf'; 'SubIndex', '24', '8', 'LE', 'unsigned', 'Standard', '0', '1', '0', '-Inf', 'Inf' }  IDPort=off  TimestampPort=off  ErrorPort=off  RemotePort=off  LengthPort=off  StatusPort=off  ApplyMinMax=off
  txSDO1 : canmsglib/CAN Unpack  MsgList=(none)  MsgName=CAN Msg  MsgIDType=Standard (11-bit identifier)  MsgIdentifier=1410  MsgLength=8  SignalInfo={ 'data', '32', '32', 'LE', 'signed', 'Standard', '0', '1', '0', '-Inf', 'Inf'; 'Index', '8', '16', 'LE', 'unsigned', 'Standard', '0', '1', '0', '-Inf', 'Inf'; 'SubIndex', '24', '8', 'LE', 'unsigned', 'Standard', '0', '1', '0', '-Inf', 'Inf' }  IDPort=off  TimestampPort=off  ErrorPort=off  RemotePort=off  LengthPort=off  StatusPort=off  ApplyMinMax=off
  txSDO2 : canmsglib/CAN Unpack  MsgList=(none)  MsgName=CAN Msg  MsgIDType=Standard (11-bit identifier)  MsgIdentifier=1411  MsgLength=8  SignalInfo={ 'data', '32', '32', 'LE', 'signed', 'Standard', '0', '1', '0', '-Inf', 'Inf'; 'Index', '8', '16', 'LE', 'unsigned', 'Standard', '0', '1', '0', '-Inf', 'Inf'; 'SubIndex', '24', '8', 'LE', 'unsigned', 'Standard', '0', '1', '0', '-Inf', 'Inf' }  IDPort=off  TimestampPort=off  ErrorPort=off  RemotePort=off  LengthPort=off  StatusPort=off  ApplyMinMax=off
  txSDO3 : canmsglib/CAN Unpack  MsgList=(none)  MsgName=CAN Msg  MsgIDType=Standard (11-bit identifier)  MsgIdentifier=1412  MsgLength=8  SignalInfo={ 'data', '32', '32', 'LE', 'signed', 'Standard', '0', '1', '0', '-Inf', 'Inf'; 'Index', '8', '16', 'LE', 'unsigned', 'Standard', '0', '1', '0', '-Inf', 'Inf'; 'SubIndex', '24', '8', 'LE', 'unsigned', 'Standard', '0', '1', '0', '-Inf', 'Inf' }  IDPort=off  TimestampPort=off  ErrorPort=off  RemotePort=off  LengthPort=off  StatusPort=off  ApplyMinMax=off
  SDOs : Outport
  emcy : Outport  Port=2
  NMT_state : Outport  Port=3
  status_mode_m3_m4_m5_m6 : Outport  Port=4
  PDO_m3 : Outport  Port=5
  PDO_m4 : Outport  Port=6
  PDO_m5 : Outport  Port=7
  PDO_m6 : Outport  Port=8
  wires:
  SampleTime/1 -> Terminator/1
  Bus Creator4/1 -> SDOs/1
  txSDO/3 -> Bus Creator4/3  "SDO_subIndex"
  EMCY/2 -> Terminator1/1
  EMCY/1 -> Bus Creator1/1  "error_code_m3"
  Bus Creator1/1 -> emcy/1
  HEARTBEAT/1 -> Bus Creator6/1  "NMT_state_3"
  txSDO/1 -> Bus Creator4/1  "SDO_data"
  txSDO/2 -> Bus Creator4/2  "SDO_index"
  TxPDO1/1 -> Bus Creator5/1  "statusword_3"
  TxPDO1/2 -> Bus Creator5/2  "mode_3"
  TxPDO1/3 -> Bus Creator2/1  "current_actual_3"
  TxPDO2/1 -> Bus Creator2/2  "pos_actual_3"
  TxPDO4/1 -> Bus Creator2/3  "velocity_actual_3"
  TxPDO4/2 -> Bus Creator2/4  "torque_actual_3"
  TxPDO1_m2/3 -> Bus Creator3/1  "current_actual_4"
  TxPDO4_m2/2 -> Bus Creator3/4  "torque_actual_4"
  TxPDO4_m2/1 -> Bus Creator3/3  "velocity_actual_4"
  TxPDO1_m2/2 -> Bus Creator5/4  "mode_4"
  TxPDO2_m2/1 -> Bus Creator3/2  "pos_actual_4"
  TxPDO1_m2/1 -> Bus Creator5/3  "statusword_4"
  Bus Creator2/1 -> PDO_m3/1
  Bus Creator3/1 -> PDO_m4/1
  Bus Creator5/1 -> status_mode_m3_m4_m5_m6/1
  EMCY_m2/1 -> Bus Creator1/2  "error_code_m4"
  EMCY_m2/2 -> Terminator2/1
  HEARTBEAT_m2/1 -> Bus Creator6/2  "NMT_state_4"
  Bus Creator6/1 -> NMT_state/1
  TxPDO4/3 -> Bus Creator2/5  "torque_averaged_3"
  TxPDO4_m2/3 -> Bus Creator3/5  "torque_averaged_4"
  txSDO1/1 -> Bus Creator4/4  "SDO_data2"
  txSDO1/2 -> Bus Creator4/5  "SDO_index2"
  txSDO1/3 -> Bus Creator4/6  "SDO_subIndex2"
  txSDO2/2 -> Bus Creator4/8  "SDO_index3"
  txSDO2/3 -> Bus Creator4/9  "SDO_subIndex3"
  txSDO2/1 -> Bus Creator4/7  "SDO_data3"
  EMCY_m3/2 -> Terminator3/1
  EMCY_m3/1 -> Bus Creator1/3  "error_code_m5"
  HEARTBEAT_m3/1 -> Bus Creator6/3  "NMT_state_5"
  TxPDO2_m3/1 -> Bus Creator7/2  "pos_actual_5"
  TxPDO4_m3/3 -> Bus Creator7/5  "torque_averaged_5"
  TxPDO1_m3/1 -> Bus Creator5/5  "statusword_5"
  Bus Creator7/1 -> PDO_m5/1
  TxPDO1_m3/3 -> Bus Creator7/1  "current_actual_5"
  TxPDO4_m3/1 -> Bus Creator7/3  "velocity_actual_5"
  TxPDO4_m3/2 -> Bus Creator7/4  "torque_actual_5"
  TxPDO1_m3/2 -> Bus Creator5/6  "mode_5"
  CAN Read/1 -> While Iterator/1
  txSDO3/1 -> Bus Creator4/10  "SDO_data4"
  txSDO3/2 -> Bus Creator4/11  "SDO_index4"
  txSDO3/3 -> Bus Creator4/12  "SDO_subIndex4"
  EMCY_m4/2 -> Terminator4/1
  EMCY_m4/1 -> Bus Creator1/4  "error_code_m6"
  HEARTBEAT_m4/1 -> Bus Creator6/4  "NMT_state_6"
  TxPDO2_m4/1 -> Bus Creator8/2  "pos_actual_6"
  CAN Read/2 -> EMCY_m2/1, EMCY_m3/1, TxPDO1_m4/1, TxPDO2_m4/1, TxPDO4_m4/1, TxPDO4_m3/1, TxPDO2_m3/1, TxPDO1_m3/1, TxPDO4_m2/1, TxPDO2_m2/1, TxPDO1/1, TxPDO2/1, TxPDO4/1, TxPDO1_m2/1, HEARTBEAT_m4/1, HEARTBEAT_m3/1, HEARTBEAT_m2/1, HEARTBEAT/1, EMCY_m4/1, EMCY/1, txSDO3/1, txSDO2/1, txSDO/1, txSDO1/1
  TxPDO4_m4/3 -> Bus Creator8/5  "torque_averaged_6"
  TxPDO1_m4/2 -> Bus Creator5/8  "mode_6"
  TxPDO1_m4/3 -> Bus Creator8/1  "current_actual_6"
  TxPDO4_m4/1 -> Bus Creator8/3  "velocity_actual_6"
  TxPDO4_m4/2 -> Bus Creator8/4  "torque_actual_6"
  Bus Creator8/1 -> PDO_m6/1
  TxPDO1_m4/1 -> Bus Creator5/7  "statusword_6"

== system ExoskeletonControlModel/OutputDataTX/SendPositionToEPOS ==
  note: SEND TARGET POSITION TO EPOS SERVOMOTOR CONTROLLER
  PositionsCommandsEPOS_Inc : Inport
  Demux : Demux  Outputs=6
  receive_PDO3_m1 : Subsystem
  receive_PDO3_m2 : Subsystem
  receive_PDO3_m3 : Subsystem
  receive_PDO3_m4 : Subsystem
  receive_PDO3_m5 : Subsystem
  receive_PDO3_m6 : Subsystem
  send_pos : Constant  Value=0
  wires:
  Demux/5 -> receive_PDO3_m5/1(target_pos)  "PositionCommandEPOSM5_inc"
  send_pos/1 -> receive_PDO3_m5/Enable, receive_PDO3_m6/Enable, receive_PDO3_m4/Enable, receive_PDO3_m3/Enable, receive_PDO3_m2/Enable, receive_PDO3_m1/Enable
  PositionsCommandsEPOS_Inc/1 -> Demux/1
  Demux/2 -> receive_PDO3_m2/1(target_pos)  "PositionCommandEPOSM2_inc"
  Demux/1 -> receive_PDO3_m1/1(target_pos)  "PositionCommandEPOSM1_inc"
  Demux/3 -> receive_PDO3_m3/1(target_pos)  "PositionCommandEPOSM3_inc"
  Demux/4 -> receive_PDO3_m4/1(target_pos)  "PositionCommandEPOSM4_inc"
  Demux/6 -> receive_PDO3_m6/1(target_pos)  "PositionCommandEPOSM6_inc"

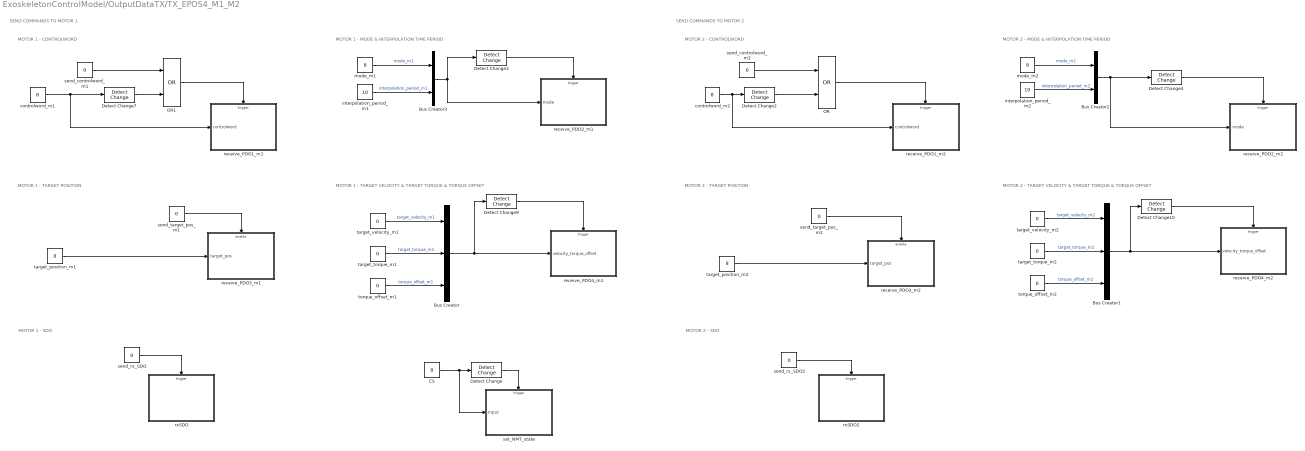
== system ExoskeletonControlModel/OutputDataTX/TX_EPOS4_M1_M2 ==
  note: MOTOR 1 - CONTROLWORD
  note: SEND COMMANDS TO MOTOR 1
  note: MOTOR 1 - TARGET VELOCITY & TARGET TORQUE & TORQUE OFFSET
  note: MOTOR 1 - MODE & INTERPOLATION TIME PERIOD
  note: MOTOR 1 - TARGET POSITION
  note: MOTOR 2 - CONTROLWORD
  note: MOTOR 2 - MODE & INTERPOLATION TIME PERIOD
  note: MOTOR 2 - TARGET POSITION
  note: MOTOR 2 - TARGET VELOCITY & TARGET TORQUE & TORQUE OFFSET
  note: SEND COMMANDS TO MOTOR 2
  note: MOTOR 2 - SDO
  note: MOTOR 1 - SDO
  Bus Creator : BusCreator  Inputs=3
  Bus Creator1 : BusCreator  Inputs=3
  Bus Creator2 : BusCreator  Inputs=2
  Bus Creator3 : BusCreator  Inputs=2
  CS : Constant  Value=8
  Detect Change{,2..4,7,9..10} (7 alike) : simulink/Logic and Bit Operations/Detect Change  vinit=0  OutDataTypeStr=boolean
  OR : Logic  Operator=OR  IconShape=distinctive  AllPortsSameDT=off  OutDataTypeStr=boolean
  OR1 : Logic  Operator=OR  IconShape=distinctive  AllPortsSameDT=off  OutDataTypeStr=boolean
  controlword_m1 : Constant  Value=8
  controlword_m2 : Constant  Value=8
  interpolation_period_m1 : Constant  Value=10
  interpolation_period_m2 : Constant  Value=10
  mode_m1 : Constant  Value=8
  mode_m2 : Constant  Value=8
  receive_PDO1_m1 : Subsystem
  receive_PDO1_m2 : Subsystem
  receive_PDO2_m1 : Subsystem
  receive_PDO2_m2 : Subsystem
  receive_PDO3_m1 : Subsystem
  receive_PDO3_m2 : Subsystem
  receive_PDO4_m1 : Subsystem
  receive_PDO4_m2 : Subsystem
  rxSDO : Subsystem
  rxSDO2 : Subsystem
  send_controlword_m1 : Constant  Value=0
  send_controlword_m2 : Constant  Value=0
  send_rx_SDO : Constant  Value=0
  send_rx_SDO2 : Constant  Value=0
  send_target_pos_m1 : Constant  Value=0
  send_target_pos_m2 : Constant  Value=0
  set_NMT_state : Subsystem
  target_position_m1 : Constant  Value=8
  target_position_m2 : Constant  Value=8
  target_torque_m1 : Constant  Value=0
  target_torque_m2 : Constant  Value=0
  target_velocity_m1 : Constant  Value=0
  target_velocity_m2 : Constant  Value=0
  torque_offset_m1 : Constant  Value=0
  torque_offset_m2 : Constant  Value=0
  wires:
  send_rx_SDO/1 -> rxSDO/Trigger
  OR1/1 -> receive_PDO1_m1/Trigger
  send_controlword_m2/1 -> OR/1
  Bus Creator3/1 -> Detect Change3/1, receive_PDO2_m1/1(mode)
  Detect Change4/1 -> receive_PDO2_m2/Trigger
  Bus Creator2/1 -> receive_PDO2_m2/1(mode), Detect Change4/1
  Detect Change3/1 -> receive_PDO2_m1/Trigger
  Detect Change10/1 -> receive_PDO4_m2/Trigger
  Detect Change2/1 -> OR/2
  OR/1 -> receive_PDO1_m2/Trigger
  controlword_m2/1 -> receive_PDO1_m2/1(controlword), Detect Change2/1
  send_controlword_m1/1 -> OR1/1
  Detect Change7/1 -> OR1/2
  controlword_m1/1 -> receive_PDO1_m1/1(controlword), Detect Change7/1
  target_position_m2/1 -> receive_PDO3_m2/1(target_pos)
  send_target_pos_m2/1 -> receive_PDO3_m2/Enable
  target_position_m1/1 -> receive_PDO3_m1/1(target_pos)
  send_target_pos_m1/1 -> receive_PDO3_m1/Enable
  Bus Creator/1 -> receive_PDO4_m1/1(velocity_torque_offset), Detect Change9/1
  Detect Change9/1 -> receive_PDO4_m1/Trigger
  target_velocity_m1/1 -> Bus Creator/1  "target_velocity_m1"
  target_torque_m1/1 -> Bus Creator/2  "target_torque_m1"
  torque_offset_m1/1 -> Bus Creator/3  "torque_offset_m1"
  target_torque_m2/1 -> Bus Creator1/2  "target_torque_m2"
  torque_offset_m2/1 -> Bus Creator1/3  "torque_offset_m2"
  target_velocity_m2/1 -> Bus Creator1/1  "target_velocity_m2"
  Bus Creator1/1 -> Detect Change10/1, receive_PDO4_m2/1(velocity_torque_offset)
  send_rx_SDO2/1 -> rxSDO2/Trigger
  Detect Change/1 -> set_NMT_state/Trigger
  CS/1 -> set_NMT_state/1(Input), Detect Change/1
  mode_m2/1 -> Bus Creator2/1  "mode_m2"
  interpolation_period_m2/1 -> Bus Creator2/2  "interpolation_period_m2"
  mode_m1/1 -> Bus Creator3/1  "mode_m1"
  interpolation_period_m1/1 -> Bus Creator3/2  "interpolation_period_m1"

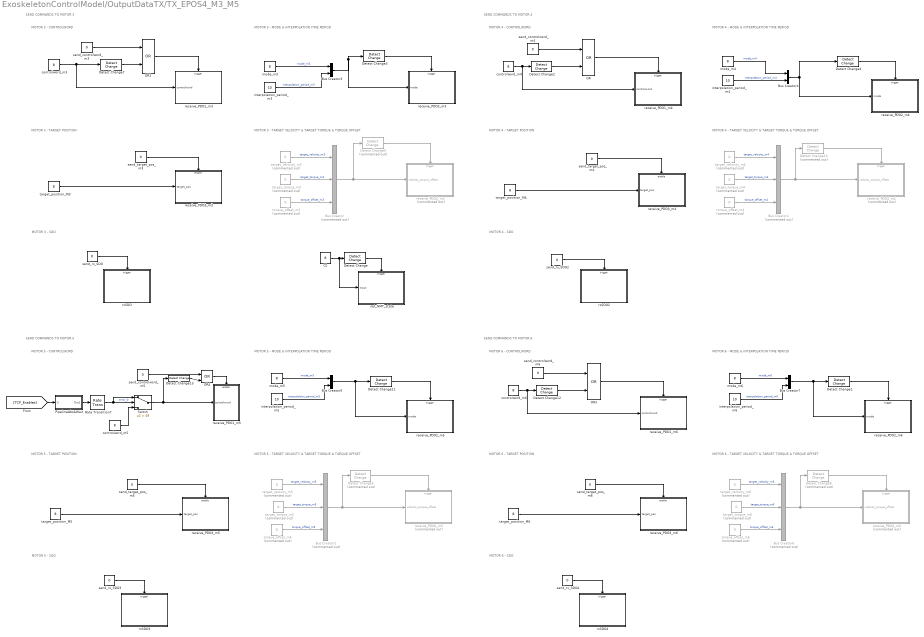
== system ExoskeletonControlModel/OutputDataTX/TX_EPOS4_M3_M5 ==
  note: MOTOR 3 - SDO
  note: MOTOR 3 - MODE & INTERPOLATION TIME PERIOD
  note: MOTOR 3 - TARGET POSITION
  note: SEND COMMANDS TO MOTOR 3
  note: MOTOR 3 - TARGET VELOCITY & TARGET TORQUE & TORQUE OFFSET
  note: MOTOR 3 - CONTROLWORD
  note: MOTOR 4 - SDO
  note: MOTOR 4 - MODE & INTERPOLATION TIME PERIOD
  note: MOTOR 4 - TARGET POSITION
  note: SEND COMMANDS TO MOTOR 4
  note: MOTOR 4 - TARGET VELOCITY & TARGET TORQUE & TORQUE OFFSET
  note: MOTOR 4 - CONTROLWORD
  note: MOTOR 5 - SDO
  note: MOTOR 5 - MODE & INTERPOLATION TIME PERIOD
  note: MOTOR 5 - TARGET POSITION
  note: SEND COMMANDS TO MOTOR 5
  note: MOTOR 5 - TARGET VELOCITY & TARGET TORQUE & TORQUE OFFSET
  note: MOTOR 5 - CONTROLWORD
  note: MOTOR 6 - SDO
  note: MOTOR 6 - TARGET POSITION
  note: SEND COMMANDS TO MOTOR 6
  note: MOTOR 6 - TARGET VELOCITY & TARGET TORQUE & TORQUE OFFSET
  note: MOTOR 6 - CONTROLWORD
  note: MOTOR 6 - MODE & INTERPOLATION TIME PERIOD
  Bus Creator{,1..2,6} (4 alike) : BusCreator  Commented=on  Inputs=3
  Bus Creator{3..5,7} (4 alike) : BusCreator  Inputs=2
  CS : Constant  Value=8
  Detect Change{,1..4,7,11..13} (9 alike) : simulink/Logic and Bit Operations/Detect Change  vinit=0  OutDataTypeStr=boolean
  Detect Change{5,8..10} (4 alike) : simulink/Logic and Bit Operations/Detect Change  Commented=on  vinit=0  OutDataTypeStr=boolean
  OR{,1,3..4} (4 alike) : Logic  Operator=OR  IconShape=distinctive  AllPortsSameDT=off  OutDataTypeStr=boolean
  PipelineAbs&Wait : Subsystem
  Rate Transition7 : RateTransition  Deterministic=off  OutPortSampleTime=Ts
  Switch : Switch  Criteria=u2 > Threshold  Threshold=49  SaturateOnIntegerOverflow=off  InputSameDT=off
  controlword_m{3..6} (4 alike) : Constant  Value=8
  interpolation_period_m{3..6} (4 alike) : Constant  Value=10
  mode_m{3..6} (4 alike) : Constant  Value=8
  receive_PDO1_m3 : Subsystem
  receive_PDO1_m4 : Subsystem
  receive_PDO1_m5 : Subsystem
  receive_PDO1_m6 : Subsystem
  receive_PDO2_m3 : Subsystem
  receive_PDO2_m4 : Subsystem
  receive_PDO2_m5 : Subsystem
  receive_PDO2_m6 : Subsystem
  receive_PDO3_m3 : Subsystem
  receive_PDO3_m4 : Subsystem
  receive_PDO3_m5 : Subsystem
  receive_PDO3_m6 : Subsystem
  receive_PDO4_m3 : Subsystem  Commented=on
  receive_PDO4_m4 : Subsystem  Commented=on
  receive_PDO4_m5 : Subsystem  Commented=on
  receive_PDO4_m6 : Subsystem  Commented=on
  rxSDO : Subsystem
  rxSDO2 : Subsystem
  rxSDO3 : Subsystem
  rxSDO4 : Subsystem
  send_controlword_m{3..6} (4 alike) : Constant  Value=0
  send_rx_SDO{,2..4} (4 alike) : Constant  Value=0
  send_target_pos_m{3..6} (4 alike) : Constant  Value=0
  set_NMT_state : Subsystem
  target_position_M{3..6} (4 alike) : Constant  Value=8
  target_torque_m{3..6} (4 alike) : Constant  Commented=on  Value=0
  target_velocity_m{3..6} (4 alike) : Constant  Commented=on  Value=0
  torque_offset_m{3..6} (4 alike) : Constant  Commented=on  Value=0
  wires:
  send_rx_SDO/1 -> rxSDO/Trigger
  OR1/1 -> receive_PDO1_m3/Trigger
  send_controlword_m4/1 -> OR/1
  Bus Creator3/1 -> receive_PDO2_m3/1(mode), Detect Change3/1
  Detect Change4/1 -> receive_PDO2_m4/Trigger
  Bus Creator4/1 -> Detect Change4/1, receive_PDO2_m4/1(mode)
  Detect Change3/1 -> receive_PDO2_m3/Trigger
  Detect Change10/1 -> receive_PDO4_m4/Trigger
  Detect Change2/1 -> OR/2
  OR/1 -> receive_PDO1_m4/Trigger
  controlword_m4/1 -> receive_PDO1_m4/1(controlword), Detect Change2/1
  send_controlword_m3/1 -> OR1/1
  Detect Change7/1 -> OR1/2
  controlword_m3/1 -> receive_PDO1_m3/1(controlword), Detect Change7/1
  target_position_M4/1 -> receive_PDO3_m4/1(target_pos)
  send_target_pos_m4/1 -> receive_PDO3_m4/Enable
  target_position_M3/1 -> receive_PDO3_m3/1(target_pos)
  send_target_pos_m3/1 -> receive_PDO3_m3/Enable
  Bus Creator/1 -> receive_PDO4_m3/1(velocity_torque_offset), Detect Change9/1
  Detect Change9/1 -> receive_PDO4_m3/Trigger
  target_velocity_m3/1 -> Bus Creator/1  "target_velocity_m3"
  target_torque_m3/1 -> Bus Creator/2  "target_torque_m3"
  torque_offset_m3/1 -> Bus Creator/3  "torque_offset_m3"
  target_torque_m4/1 -> Bus Creator1/2  "target_torque_m4"
  torque_offset_m4/1 -> Bus Creator1/3  "torque_offset_m4"
  target_velocity_m4/1 -> Bus Creator1/1  "target_velocity_m4"
  Bus Creator1/1 -> Detect Change10/1, receive_PDO4_m4/1(velocity_torque_offset)
  send_rx_SDO2/1 -> rxSDO2/Trigger
  send_rx_SDO3/1 -> rxSDO3/Trigger
  Detect Change11/1 -> receive_PDO2_m5/Trigger
  target_velocity_m5/1 -> Bus Creator2/1  "target_velocity_m5"
  torque_offset_m5/1 -> Bus Creator2/3  "torque_offset_m5"
  target_position_M5/1 -> receive_PDO3_m5/1(target_pos)
  target_torque_m5/1 -> Bus Creator2/2  "target_torque_m5"
  Bus Creator2/1 -> Detect Change5/1, receive_PDO4_m5/1(velocity_torque_offset)
  Detect Change5/1 -> receive_PDO4_m5/Trigger
  send_target_pos_m5/1 -> receive_PDO3_m5/Enable
  Bus Creator5/1 -> receive_PDO2_m5/1(mode), Detect Change11/1
  Detect Change/1 -> set_NMT_state/Trigger
  CS/1 -> set_NMT_state/1(Input), Detect Change/1
  interpolation_period_m3/1 -> Bus Creator3/2  "interpolation_period_m3"
  mode_m3/1 -> Bus Creator3/1  "mode_m3"
  interpolation_period_m4/1 -> Bus Creator4/2  "interpolation_period_m4"
  mode_m4/1 -> Bus Creator4/1  "mode_m4"
  mode_m5/1 -> Bus Creator5/1  "mode_m5"
  interpolation_period_m5/1 -> Bus Creator5/2  "interpolation_period_m5"
  OR3/1 -> receive_PDO1_m6/Trigger
  Bus Creator7/1 -> receive_PDO2_m6/1(mode), Detect Change1/1
  Detect Change12/1 -> OR3/2
  target_velocity_m6/1 -> Bus Creator6/1  "target_velocity_m6"
  Detect Change8/1 -> receive_PDO4_m6/Trigger
  send_controlword_m6/1 -> OR3/1
  Bus Creator6/1 -> Detect Change8/1, receive_PDO4_m6/1(velocity_torque_offset)
  target_torque_m6/1 -> Bus Creator6/2  "target_torque_m6"
  Detect Change1/1 -> receive_PDO2_m6/Trigger
  torque_offset_m6/1 -> Bus Creator6/3  "torque_offset_m6"
  controlword_m6/1 -> receive_PDO1_m6/1(controlword), Detect Change12/1
  send_rx_SDO4/1 -> rxSDO4/Trigger
  send_target_pos_m6/1 -> receive_PDO3_m6/Enable
  mode_m6/1 -> Bus Creator7/1  "mode_m6"
  target_position_M6/1 -> receive_PDO3_m6/1(target_pos)
  interpolation_period_m6/1 -> Bus Creator7/2  "interpolation_period_m6"
  Switch/1 -> receive_PDO1_m5/1(controlword), Detect Change13/1
  Rate Transition7/1 -> Switch/1, Switch/2  "error_0"
  PipelineAbs&Wait/1(Out1) -> Rate Transition7/1
  send_controlword_m5/1 -> OR4/1
  controlword_m5/1 -> Switch/3
  OR4/1 -> receive_PDO1_m5/Enable
  [TCP_Enables] -> PipelineAbs&Wait/1(U)
  Detect Change13/1 -> OR4/2

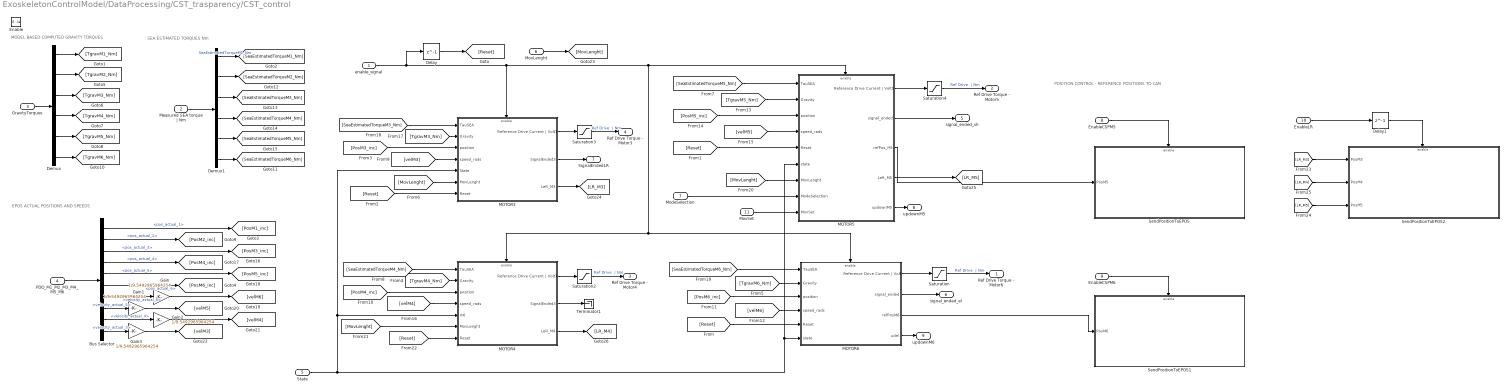
== system ExoskeletonControlModel/DataProcessing/CST_trasparency/CST_control ==
  note: POSITION CONTROL - REFERENCE POSITIONS TO CAN
  note: EPOS ACTUAL POSITIONS AND SPEEDS
  note: MODEL BASED COMPUTED GRAVITY TORQUES
  note: SEA ESTIMATED TORQUES Nm
  enable_signal : Inport
  Measured SEA torque | Nm : Inport  Port=2
  GravityTorques : Inport  Port=3
  PDO_M1_M2_M3_M4_M5_M6 : Inport  Port=4
  State : Inport  Port=5
  MovLenght : Inport  Port=6
  ModeSelection : Inport  Port=7
  EnableCSPM5 : Inport  Port=8
  EnableCSPM6 : Inport  Port=9
  EnableLR : Inport  Port=10
  MovSet : Inport  Port=11
  Enable : EnablePort
  Bus Selector : BusSelector  OutputSignals=PDO_M1.pos_actual_1,PDO_M2.pos_actual_2,PDO_M3.pos_actual_3,PDO_M4.pos_actual_4,PDO_M5.pos_actual_5,PDO_M6.pos_actual_6,PDO_M6.velocity_actual_6,PDO_M5.velocity_actual_5,PDO_M4.velocity_actual_4,PDO_M3.velocity_actual_3
  Delay : Delay  DelayLength=1
  Delay1 : Delay  DelayLength=1
  Demux : Demux  Outputs=6
  Demux1 : Demux  Outputs=6
  Gain{,1..3} (4 alike) : Gain  Gain=1/9.5492965964254
  MOTOR3 : Subsystem
  MOTOR4 : Subsystem
  MOTOR5 : Subsystem
  MOTOR6 : Subsystem
  Saturation{,2..4} (4 alike) : Saturate  UpperLimit=1000  LowerLimit=-1000
  SendPositionToEPOS : Subsystem
  SendPositionToEPOS1 : Subsystem
  SendPositionToEPOS2 : Subsystem
  Terminator1 : Terminator
  Ref Drive Torque - Motor6 : Outport
  Ref Drive Torque - Motor5 : Outport  Port=2
  Ref Drive Torque - Motor4 : Outport  Port=3
  Ref Drive Torque - Motor3 : Outport  Port=4
  signal_ended_sh : Outport  Port=5  InitialOutput=0
  signal_ended_el : Outport  Port=6  InitialOutput=0
  SignalEndedLR : Outport  Port=7  InitialOutput=0
  updownM5 : Outport  Port=8  InitialOutput=0
  updownM6 : Outport  Port=9  InitialOutput=0
  wires:
  enable_signal/1 -> Delay/1, MOTOR6/Enable, MOTOR4/Enable, MOTOR5/Enable, MOTOR3/Enable
  MOTOR6/1(Reference Drive Current | Volt) -> Saturation/1
  Demux1/3 -> [SeaEstimatedTorqueM3_Nm]
  Demux1/2 -> [SeaEstimatedTorqueM2_Nm]
  Demux1/5 -> [SeaEstimatedTorqueM5_Nm]
  Demux1/4 -> [SeaEstimatedTorqueM4_Nm]
  Demux1/6 -> [SeaEstimatedTorqueM6_Nm]
  Measured SEA torque | Nm/1 -> Demux1/1
  Demux1/1 -> [SeaEstimatedTorqueM1_Nm]  "SeaEstimatedTorqueM1_Nm"
  Saturation/1 -> Ref Drive Torque - Motor6/1  "Ref Drive  | Nm"
  Saturation4/1 -> Ref Drive Torque - Motor5/1  "Ref Drive  | Nm"
  MOTOR4/1(Reference Drive Current | Volt1) -> Saturation2/1
  Saturation2/1 -> Ref Drive Torque - Motor4/1  "Ref Drive  | Nm"
  Saturation3/1 -> Ref Drive Torque - Motor3/1  "Ref Drive  | Nm"
  MOTOR3/1(Reference Drive Current | Volt1) -> Saturation3/1
  [TgravM6_Nm] -> MOTOR6/2(Gravity)
  Demux/3 -> [TgravM3_Nm]
  Demux/4 -> [TgravM4_Nm]
  Demux/2 -> [TgravM2_Nm]
  Demux/1 -> [TgravM1_Nm]
  Demux/5 -> [TgravM5_Nm]
  GravityTorques/1 -> Demux/1
  Demux/6 -> [TgravM6_Nm]
  PDO_M1_M2_M3_M4_M5_M6/1 -> Bus Selector/1
  Bus Selector/1 -> [PosM1_inc]  "<pos_actual_1>"
  Bus Selector/2 -> [PosM2_inc]  "<pos_actual_2>"
  Bus Selector/3 -> [PosM3_inc]  "<pos_actual_3>"
  Bus Selector/4 -> [PosM4_inc]  "<pos_actual_4>"
  Bus Selector/5 -> [PosM5_inc]  "<pos_actual_5>"
  Bus Selector/6 -> [PosM6_inc]  "<pos_actual_6>"
  [PosM6_inc] -> MOTOR6/3(position)
  Bus Selector/7 -> Gain/1  "<velocity_actual_6>"
  Gain/1 -> [velM6]
  [velM6] -> MOTOR6/4(speed_rads)
  Gain1/1 -> [velM5]
  Bus Selector/8 -> Gain1/1  "<velocity_actual_5>"
  Gain2/1 -> [velM4]
  Bus Selector/9 -> Gain2/1  "<velocity_actual_4>"
  Gain3/1 -> [velM3]
  Bus Selector/10 -> Gain3/1  "<velocity_actual_3>"
  [TgravM5_Nm] -> MOTOR5/2(Gravity)
  [PosM5_inc] -> MOTOR5/3(position)
  [velM5] -> MOTOR5/4(speed_rads)
  MOTOR5/1(Reference Drive Current | Volt1) -> Saturation4/1
  [TgravM4_Nm] -> MOTOR4/2(Gravity)
  [velM4] -> MOTOR4/4(speed_rads)
  [PosM4_inc] -> MOTOR4/3(position)
  [TgravM3_Nm] -> MOTOR3/2(Gravity)
  [PosM3_inc] -> MOTOR3/3(position)
  [velM3] -> MOTOR3/4(speed_rads)
  [Reset] -> MOTOR6/5(Reset)
  [SeaEstimatedTorqueM5_Nm] -> MOTOR5/1(TauSEA)
  [SeaEstimatedTorqueM4_Nm] -> MOTOR4/1(TauSEA)
  [SeaEstimatedTorqueM3_Nm] -> MOTOR3/1(TauSEA)
  [SeaEstimatedTorqueM6_Nm] -> MOTOR6/1(TauSEA)
  [Reset] -> MOTOR5/5(Reset)
  Delay/1 -> [Reset]
  MOTOR5/2(signal_ended) -> signal_ended_sh/1
  State/1 -> MOTOR6/6(state), MOTOR5/6(state), MOTOR4/5(In6), MOTOR3/5(State)
  MOTOR6/2(signal_ended) -> signal_ended_el/1
  ModeSelection/1 -> MOTOR5/8(ModeSelection)
  [Reset] -> MOTOR3/7(Reset)
  MOTOR3/2(SignalEnded3) -> SignalEndedLR/1
  MovLenght/1 -> [MovLenght]
  [MovLenght] -> MOTOR3/6(MovLenght)
  [MovLenght] -> MOTOR5/7(MovLenght)
  [MovLenght] -> MOTOR4/6(MovLenght)
  [Reset] -> MOTOR4/7(Reset)
  MOTOR4/2(SignalEnded3) -> Terminator1/1
  MOTOR5/3(refPos_M5) -> SendPositionToEPOS/1(PosM5)
  MOTOR6/3(refPosM6) -> SendPositionToEPOS1/1(PosM6)
  EnableCSPM5/1 -> SendPositionToEPOS/Enable
  EnableCSPM6/1 -> SendPositionToEPOS1/Enable
  EnableLR/1 -> Delay1/1
  MOTOR3/3(LeR_M3) -> [LR_M3]
  MOTOR5/4(LeR_M5) -> [LR_M5]
  MOTOR4/3(LeR_M4) -> [LR_M4]
  [LR_M3] -> SendPositionToEPOS2/1(PosM3)
  [LR_M4] -> SendPositionToEPOS2/2(PosM4)
  [LR_M5] -> SendPositionToEPOS2/3(PosM5)
  Delay1/1 -> SendPositionToEPOS2/Enable
  MovSet/1 -> MOTOR5/9(MovSet)
  MOTOR5/5(updownM5) -> updownM5/1
  MOTOR6/4(udel) -> updownM6/1
